simulink model "spike_detection"  (R2018b)
settings: Solver=FixedStepDiscrete  StartTime=0.0  StopTime=10.0  RelTol=1e-3  EnableMultiTasking=on
libraries: simulink x12, dspswit3 x1, hdlsllib x1, dspbuff3 x1
settings Model: Creator=diyar  LastModifiedBy=diyar
settings SolverCC: AutoInsertRateTranBlk=on
settings DebuggingCC: SingleTaskRateTransMsg=error

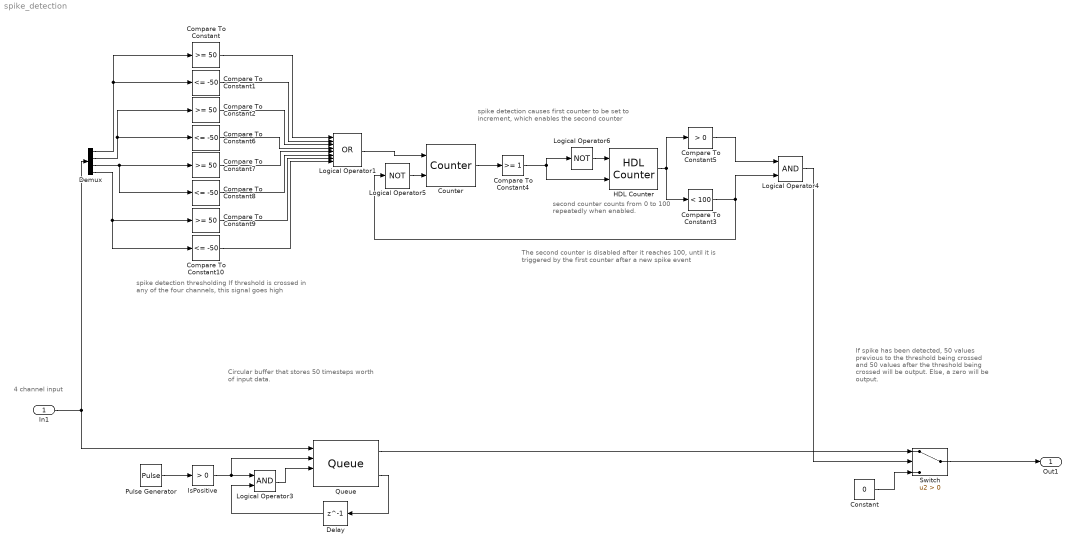
== system spike_detection ==
  note: If spike has been detected, 50 values previous to the threshold being crossed and 50 values after the threshold being crossed will be output. Else, a zero will be output.
  note: The second counter is disabled after it reaches 100, until it is triggered by the first counter after a new spike event
  note: Circular buffer that stores 50 timesteps worth of input data.
  note: second counter counts from 0 to 100 repeatedly when enabled.
  note: spike detection causes first counter to be set to increment, which enables the second counter
  note: spike detection thresholding
      | If threshold is crossed in any of the four channels, this signal goes high
  note: 4 channel input
  In1 : Inport  OutDataTypeStr=double  PortDimensions=4  SampleTime=1
  Compare To Constant{,2,7,9} (4 alike) : simulink/Logic and Bit Operations/Compare To Constant  relop=>=  const=50  OutDataTypeStr=boolean
  Compare To Constant{1,6,8,10} (4 alike) : simulink/Logic and Bit Operations/Compare To Constant  relop=<=  const=-50  OutDataTypeStr=boolean
  Compare To Constant3 : simulink/Logic and Bit Operations/Compare To Constant  relop=<  const=100  OutDataTypeStr=boolean
  Compare To Constant4 : simulink/Logic and Bit Operations/Compare To Constant  relop=>=  const=1  OutDataTypeStr=boolean
  Compare To Constant5 : simulink/Logic and Bit Operations/Compare To Constant  relop=>  const=0  OutDataTypeStr=boolean
  Constant : Constant  Value=0  SampleTime=1
  Counter : dspswit3/Counter  Direction=Up  CountEvent=Rising edge  CounterSize=8 bits  MaxCount=1  InitialCount=0  Output=Count  HitValue=1  ResetInput=on  SamplesPerFrame=1  Ts=1  CntDtype=uint8  HitDtype=Boolean
  Delay : Delay  DelayLength=1  InitialCondition=0
  Demux : Demux
  HDL Counter : hdlsllib/Sources/HDL Counter  CountType=Count limited  CountInit=0  CountStep=1  CountMax=100  CountFromType=Initial value  CountFrom=0  CountResetPort=on  CountLoadPort=off  CountEnbPort=on  CountDirPort=off  CountDataType=Unsigned  CountWordLen=20  CountFracLen=0  CountSampTime=1
      settings: SourceProductBaseCode=HD
  IsPositive : simulink/Logic and Bit Operations/Compare To Zero  relop=>  OutDataTypeStr=boolean
  Logical Operator1 : Logic  Operator=OR  Inputs=8  AllPortsSameDT=off  OutDataTypeStr=boolean
  Logical Operator3 : Logic  OutDataTypeStr=boolean
  Logical Operator4 : Logic  AllPortsSameDT=off  OutDataTypeStr=boolean
  Logical Operator5 : Logic  Operator=NOT  AllPortsSameDT=off  OutDataTypeStr=boolean
  Logical Operator6 : Logic  Operator=NOT  AllPortsSameDT=off  OutDataTypeStr=boolean
  Pulse Generator : DiscretePulseGenerator
  Queue : dspbuff3/Queue  depth=50  trigger=Either edge  overflow=Ignore  pes=Warning  eso=off  fso=on  nso=off  clr=on  clrOutport=off  adf=off
      settings: SourceProductName=DSP System Toolbox  SourceProductBaseCode=DS
  Switch : Switch  Criteria=u2 > Threshold
  Out1 : Outport
  wires:
  Compare To Constant/1 -> Logical Operator1/1
  Compare To Constant1/1 -> Logical Operator1/2
  Switch/1 -> Out1/1
  Constant/1 -> Switch/3
  Logical Operator3/1 -> Queue/3
  Queue/2 -> Delay/1
  Pulse Generator/1 -> IsPositive/1
  Delay/1 -> Logical Operator3/2
  IsPositive/1 -> Queue/2, Logical Operator3/1
  HDL Counter/1 -> Compare To Constant5/1, Compare To Constant3/1
  Compare To Constant5/1 -> Logical Operator4/1
  Compare To Constant3/1 -> Logical Operator5/1, Logical Operator4/2
  Logical Operator1/1 -> Counter/1
  Logical Operator4/1 -> Switch/2
  In1/1 -> Queue/1, Demux/1
  Demux/1 -> Compare To Constant/1, Compare To Constant1/1
  Compare To Constant6/1 -> Logical Operator1/4
  Compare To Constant2/1 -> Logical Operator1/3
  Demux/2 -> Compare To Constant6/1, Compare To Constant2/1
  Compare To Constant8/1 -> Logical Operator1/6
  Compare To Constant7/1 -> Logical Operator1/5
  Compare To Constant9/1 -> Logical Operator1/7
  Demux/3 -> Compare To Constant8/1, Compare To Constant7/1
  Demux/4 -> Compare To Constant10/1, Compare To Constant9/1
  Compare To Constant10/1 -> Logical Operator1/8
  Queue/1 -> Switch/1
  Logical Operator6/1 -> HDL Counter/1
  Compare To Constant4/1 -> HDL Counter/2, Logical Operator6/1
  Counter/1 -> Compare To Constant4/1
  Logical Operator5/1 -> Counter/2
